simulink library "se2a_environment_lib"  (R2018b)
settings: Solver=VariableStepAuto  StartTime=0.0  StopTime=10.0  RelTol=1e-3
undefined symbols (not defined in the file or in its folder): aircraft, alt_ground, atmosphere, Atmosphere, cntrl, envir, g, ic, pos_ref, wind
libraries: simulink x9, atmosphere_lib x6, linear_systems_lib x6, $bdroot x5
(part 1 of 2)
settings Model: Creator=Ybeyer  LastModifiedBy=yannic
settings SFSimCC: SimUseLocalCustomCode=off
settings RTWCC: RTWUseLocalCustomCode=off
settings CodeAppCC: StateflowObjectComments=on

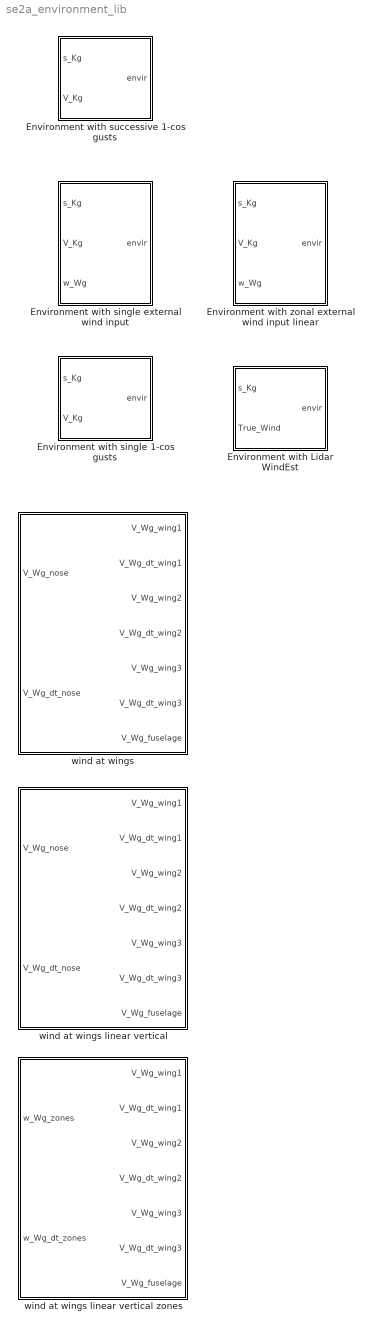
== system se2a_environment_lib ==
  Environment with Lidar WindEst : Subsystem  mask{envir=envir, pos_ref=pos_ref}
      mask prompts: envir "environment struct"; pos_ref "reference position struct"
      mask DialogControl DescGroupVar Prompt: Environment with successive 1-cos gusts
      mask DialogControl DescTextVar Prompt: Note that for the local gust delays the following structs must be in the base workspace: wing_main, wing_htp, wing_vtp, fuselage
  Environment with single 1-cos gusts : Subsystem  mask{envir=envir, pos_ref=pos_ref, wind_input=cntrl.wind_input, U_ds=-1, gust_dir=0, F_g=30, gustGradDist=30, Delta_gustGradDist=10, Delta_time=3, time_0=5}
      mask prompts: envir "environment struct"; pos_ref "reference position struct"; wind_input "Switch wing model (1=disable, 2=1-cos gust)"; U_ds "U_ds (Positive values only, if -1 value is calculated internally)"; gust_dir "Gust direction (>0 up, <0 down)"; F_g "Flight profile alleviation factor"; gustGradDist "Initial gust gradient distance, in ft"; Delta_gustGradDist "Delta gust gradient distance, in ft"; Delta_time "Time between gusts, in s"; time_0 "Time of first gust, in s"
      mask DialogControl DescGroupVar Prompt: Environment with successive 1-cos gusts
      mask DialogControl DescTextVar Prompt: Note that for the local gust delays the following structs must be in the base workspace: wing_main, wing_htp, wing_vtp, fuselage
  Environment with single external wind input : Subsystem  mask{aircraft=aircraft, V_A=norm(ic.V_Kb,2), pos_ref=pos_ref, k_max=1}
      mask prompts: aircraft "Aircraft parameters sturct, see aircraftSe2aCreate"; V_A "Airspeed (TAS) in m/s"; pos_ref "Reference position, see loadPosRef"; k_max "Wind derivative cutoff reduced frequency, rad"
      mask DialogControl DescGroupVar Prompt: Environment with single external wind input
      mask DialogControl Container2 Prompt: Parameters
  Environment with successive 1-cos gusts : Subsystem  mask{envir=envir, pos_ref=pos_ref, wind_input=cntrl.wind_input, F_g=1, gustGradDist=30, Delta_gustGradDist=10, Delta_time=3, time_0=5}
      mask prompts: envir "environment struct"; pos_ref "reference position struct"; wind_input "Switch wing model (1=disable, 2=1-cos gust)"; F_g "Flight profile alleviation factor"; gustGradDist "Initial gust gradient distance, in ft"; Delta_gustGradDist "Delta gust gradient distance, in ft"; Delta_time "Time between gusts, in s"; time_0 "Time of first gust, in s"
      mask DialogControl DescGroupVar Prompt: Environment with successive 1-cos gusts
      mask DialogControl DescTextVar Prompt: Note that for the local gust delays the following structs must be in the base workspace: wing_main, wing_htp, wing_vtp, fuselage
  Environment with zonal external wind input linear : Subsystem  mask{aircraft=aircraft, V_A=norm(ic.V_Kb,2), pos_ref=pos_ref, k_max=1}
      mask prompts: aircraft "Aircraft parameters sturct, see aircraftSe2aCreate"; V_A "Airspeed (TAS) in m/s"; pos_ref "Reference position, see loadPosRef"; k_max "Wind derivative cutoff reduced frequency, rad"
      mask DialogControl DescGroupVar Prompt: Environment with single external wind input
      mask DialogControl Container2 Prompt: Parameters
  wind at wings : Subsystem  mask{aircraft=aircraft, V_A=norm(ic.V_Kb,2)}
      mask prompts: aircraft "Aircraft parameters struct, see aircraftSe2aCreate"; V_A "Airspeed (TAS) in m/s"
      mask init:
      | Delta_time_main_wing = abs(aircraft.wing_main.params.x+aircraft.wing_main.geometry.ctrl_pt.pos(1,:))/V_A;
      | Delta_time_htp = abs(aircraft.wing_htp.params.x+aircraft.wing_htp.geometry.ctrl_pt.pos(1,:))/V_A;
      | Delta_time_vtp = abs(aircraft.wing_vtp.params.x+aircraft.wing_vtp.geometry.ctrl_pt.pos(1,:))/V_A;
      | Delta_time_fuse = abs(aircraft.fuselage.geometry.border_pos(1,:))/V_A;
  wind at wings linear vertical : Subsystem  mask{aircraft=aircraft, V_A=norm(ic.V_Kb,2)}
      mask prompts: aircraft "Aircraft parameters struct, see aircraftSe2aCreate"; V_A "Airspeed (TAS) in m/s"
      mask init:
      | Delta_time_main_wing = abs(aircraft.wing_main.params.x+aircraft.wing_main.geometry.ctrl_pt.pos(1,:))/V_A;
      | Delta_time_htp = abs(aircraft.wing_htp.params.x+aircraft.wing_htp.geometry.ctrl_pt.pos(1,:))/V_A;
      | Delta_time_vtp = abs(aircraft.wing_vtp.params.x+aircraft.wing_vtp.geometry.ctrl_pt.pos(1,:))/V_A;
      | Delta_time_fuse = abs(aircraft.fuselage.geometry.border_pos(1,:))/V_A;
      | 
      | Ts = 1/100;
      | 
      | Delay_sys_main_wing = Create_LinearDelaySys(Delta_time_main_wing, Ts);
      | Delay_sys_htp = Create_LinearDelaySys(Delta_time_htp, Ts);
      | Delay_sys_vtp = Create_LinearDelaySys(Delta_time_vtp, Ts);
      | Delay_sys_fuse = Create_LinearDelaySys(Delta_time_fuse, Ts);
  wind at wings linear vertical zones : Subsystem  mask{aircraft=aircraft, V_A=norm(ic.V_Kb,2)}
      mask prompts: aircraft "Aircraft parameters struct, see aircraftSe2aCreate"; V_A "Airspeed (TAS) in m/s"
      mask init:
      | Delta_time_main_wing = abs(aircraft.wing_main.params.x+aircraft.wing_main.geometry.ctrl_pt.pos(1,:))/V_A;
      | Delta_time_htp = abs(aircraft.wing_htp.params.x+aircraft.wing_htp.geometry.ctrl_pt.pos(1,:))/V_A;
      | Delta_time_vtp = abs(aircraft.wing_vtp.params.x+aircraft.wing_vtp.geometry.ctrl_pt.pos(1,:))/V_A;
      | Delta_time_fuse = abs(aircraft.fuselage.geometry.border_pos(1,:))/V_A;
      | 
      | Ts = 0;%1/100;
      | 
      | Delay_sys_main_wing = Create_LinearDelaySys(Delta_time_main_wing, Ts);
      | Delay_sys_htp = Create_LinearDelaySys(Delta_time_htp, Ts);
      | Delay_sys_vtp = Create_LinearDelaySys(Delta_time_vtp, Ts);
      | Delay_sys_fuse = Create_LinearDelaySys(Delta_time_fuse, Ts);

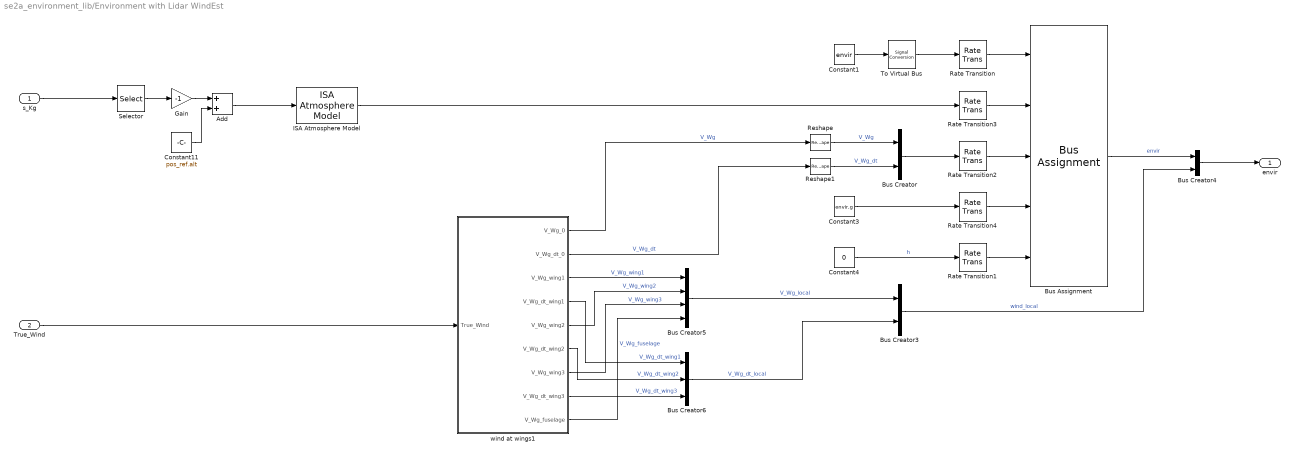
== system se2a_environment_lib/Environment with Lidar WindEst ==
  s_Kg : Inport
  True_Wind : Inport  Port=2
  Add : Sum
  Bus Assignment : BusAssignment  AssignedSignals=atmosphere,wind,g,alt_ground
  Bus Creator : BusCreator  Inputs=2
  Bus Creator3 : BusCreator  Inputs=2
  Bus Creator4 : BusCreator  Inputs=2
  Bus Creator5 : BusCreator  Inputs=4
  Bus Creator6 : BusCreator  Inputs=3
  Constant1 : Constant  Value=envir  OutDataTypeStr=Bus: envirBus
  Constant11 : Constant  Value=pos_ref.alt
  Constant3 : Constant  Value=envir.g
  Constant4 : Constant  Value=0
  Gain : Gain  Gain=-1
  ISA Atmosphere Model : atmosphere_lib/ISA Atmosphere Model
      settings: SourceProductName=LADAC
  Rate Transition{,1..4} (5 alike) : RateTransition
  Reshape : Reshape  OutputDimensionality=Column vector (2-D)
  Reshape1 : Reshape  OutputDimensionality=Column vector (2-D)
  Selector : Selector  InputPortWidth=3  IndexOptions=Index vector (dialog)  Indices=3  OutputSizes=1
  To Virtual Bus : SignalConversion  ConversionOutput=Virtual bus  OverrideOpt=off
  wind at wings1 : Subsystem  mask{aircraft=aircraft}
      mask prompts: aircraft "Aircraft parameters struct, see aircraftSe2aCreate"
      mask init:
      | n_origin = 6;
      | n_wing = aircraft.wing_main.n_panel;
      | n_htp = aircraft.wing_htp.n_panel;
      | n_vtp = aircraft.wing_vtp.n_panel;
      | n_fus = aircraft.fuselage.n_segments+1;
  envir : Outport
  wires:
  Constant4/1 -> Rate Transition1/1  "h"
  Rate Transition2/1 -> Bus Assignment/3
  Rate Transition3/1 -> Bus Assignment/2
  Bus Assignment/1 -> Bus Creator4/1  "envir"
  Rate Transition/1 -> Bus Assignment/1
  ISA Atmosphere Model/1 -> Rate Transition3/1
  Rate Transition1/1 -> Bus Assignment/5
  Constant1/1 -> To Virtual Bus/1
  Add/1 -> ISA Atmosphere Model/1
  Bus Creator/1 -> Rate Transition2/1
  wind at wings1/2(V_Wg_dt_0) -> Reshape1/1  "V_Wg_dt"
  Rate Transition4/1 -> Bus Assignment/4
  Constant3/1 -> Rate Transition4/1
  wind at wings1/1(V_Wg_0) -> Reshape/1  "V_Wg"
  Bus Creator6/1 -> Bus Creator3/2  "V_Wg_dt_local"
  Bus Creator3/1 -> Bus Creator4/2  "wind_local"
  Bus Creator4/1 -> envir/1
  To Virtual Bus/1 -> Rate Transition/1
  Constant11/1 -> Add/2
  Gain/1 -> Add/1
  s_Kg/1 -> Selector/1
  Selector/1 -> Gain/1
  True_Wind/1 -> wind at wings1/1(True_Wind)
  wind at wings1/8(V_Wg_dt_wing3) -> Bus Creator6/3  "V_Wg_dt_wing3"
  wind at wings1/6(V_Wg_dt_wing2) -> Bus Creator6/2  "V_Wg_dt_wing2"
  wind at wings1/5(V_Wg_wing2) -> Bus Creator5/2  "V_Wg_wing2"
  wind at wings1/9(V_Wg_fuselage) -> Bus Creator5/4  "V_Wg_fuselage"
  Bus Creator5/1 -> Bus Creator3/1  "V_Wg_local"
  wind at wings1/4(V_Wg_dt_wing1) -> Bus Creator6/1  "V_Wg_dt_wing1"
  wind at wings1/3(V_Wg_wing1) -> Bus Creator5/1  "V_Wg_wing1"
  wind at wings1/7(V_Wg_wing3) -> Bus Creator5/3  "V_Wg_wing3"
  Reshape/1 -> Bus Creator/1  "V_Wg"
  Reshape1/1 -> Bus Creator/2  "V_Wg_dt"

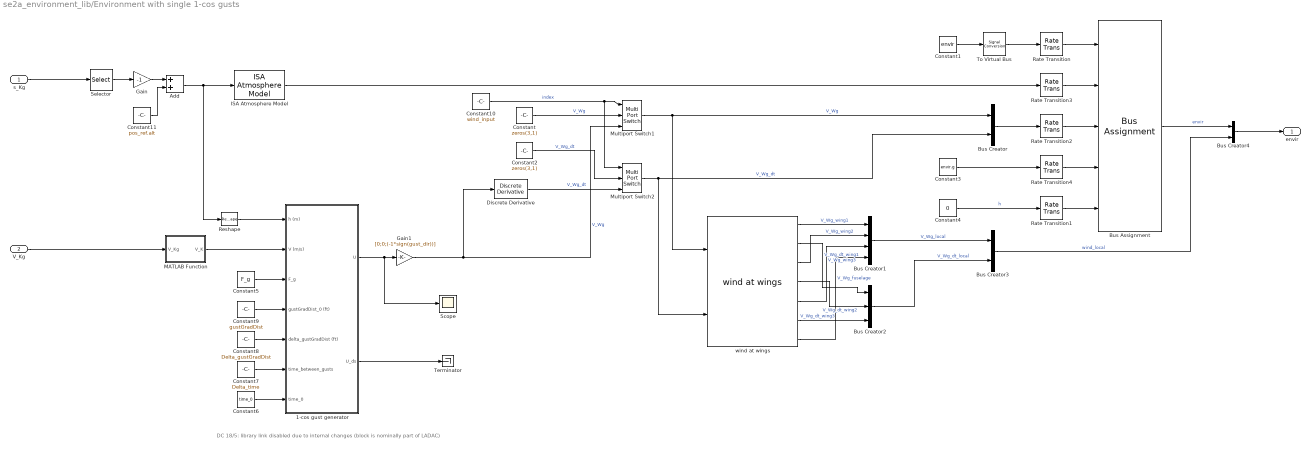
== system se2a_environment_lib/Environment with single 1-cos gusts ==
  note: DC 18/5: library link disabled due to internal changes (block is nominally part of LADAC)
  s_Kg : Inport
  V_Kg : Inport  Port=2
  1-cos gust generator : Subsystem  AncestorBlock=atmosphere_lib/1-cos gust generator
      mask DialogControl DescGroupVar Prompt: 1-cos gust generator
      mask DialogControl DescTextVar Prompt: With this block you can generate a time series of 1-cos gusts. You can use the inputs to specify parameters like the initial gust gradient distance and how you want to increment the gust gradient distance for the next gust. Moreover, you can specify the time between the gusts.
      mask DialogControl ParameterGroupVar Prompt: Inputs
      mask DialogControl Control2 Prompt: h - altitude (m)
      mask DialogControl Control3 Prompt: V - airspeed of the aircraft (m/s)
      mask DialogControl Control4 Prompt: F_g - flight profile alleviation factor
      mask DialogControl Control5 Prompt: gustGradDist_0 - initial gust gradient distance (m)
      mask DialogControl Control6 Prompt: delta_gustGradDist - difference of the gust gradient distance for the next gust (m)
      mask DialogControl Control7 Prompt: time_between gusts - the time between gusts where there will be no wind (s)
      mask DialogControl Control8 Prompt: time_0 - time when the first gust starts
  Add : Sum
  Bus Assignment : BusAssignment  AssignedSignals=atmosphere,wind,g,alt_ground
  Bus Creator : BusCreator  Inputs=2
  Bus Creator1 : BusCreator  Inputs=4
  Bus Creator2 : BusCreator  Inputs=3
  Bus Creator3 : BusCreator  Inputs=2
  Bus Creator4 : BusCreator  Inputs=2
  Constant : Constant  Value=zeros(3,1)  VectorParams1D=off
  Constant1 : Constant  Value=envir  OutDataTypeStr=Bus: envirBus
  Constant10 : Constant  Value=wind_input
  Constant11 : Constant  Value=pos_ref.alt
  Constant2 : Constant  Value=zeros(3,1)  VectorParams1D=off
  Constant3 : Constant  Value=envir.g
  Constant4 : Constant  Value=0
  Constant5 : Constant  Value=F_g
  Constant6 : Constant  Value=time_0
  Constant7 : Constant  Value=Delta_time
  Constant8 : Constant  Value=Delta_gustGradDist
  Constant9 : Constant  Value=gustGradDist
  Discrete Derivative : simulink/Discrete/Discrete Derivative  gainval=1.0  ICPrevScaledInput=0.0  OutMin=[]  OutMax=[]  OutDataType=fixdt(1, 16)  OutScaling=2^-10  DoSatur=off
  Gain : Gain  Gain=-1
  Gain1 : Gain  Gain=[0;0;(-1*sign(gust_dir))]
  ISA Atmosphere Model : atmosphere_lib/ISA Atmosphere Model
      settings: SourceProductName=LADAC
  MATLAB Function : MATLAB Function  TreatAsAtomicUnit=on
  Multiport Switch1 : MultiPortSwitch  Inputs=2
  Multiport Switch2 : MultiPortSwitch  Inputs=2
  Rate Transition{,1..4} (5 alike) : RateTransition
  Reshape : Reshape
  Scope : Scope
  Selector : Selector  InputPortWidth=3  IndexOptions=Index vector (dialog)  Indices=3  OutputSizes=1
  Terminator : Terminator
  To Virtual Bus : SignalConversion  ConversionOutput=Virtual bus  OverrideOpt=off
  wind at wings : $bdroot/wind at wings  aircraft=aircraft  V_A=norm(ic.V_Kb,2)
  envir : Outport
  wires:
  Reshape/1 -> 1-cos gust generator/1(h (m))
  wind at wings/7 -> Bus Creator1/4  "V_Wg_fuselage"
  Selector/1 -> Gain/1
  s_Kg/1 -> Selector/1
  Gain/1 -> Add/1
  Constant11/1 -> Add/2
  To Virtual Bus/1 -> Rate Transition/1
  Bus Creator4/1 -> envir/1
  Bus Creator3/1 -> Bus Creator4/2  "wind_local"
  Bus Creator2/1 -> Bus Creator3/2  "V_Wg_dt_local"
  wind at wings/2 -> Bus Creator2/1  "V_Wg_dt_wing1"
  wind at wings/4 -> Bus Creator2/2  "V_Wg_dt_wing2"
  wind at wings/6 -> Bus Creator2/3  "V_Wg_dt_wing3"
  Bus Creator1/1 -> Bus Creator3/1  "V_Wg_local"
  wind at wings/5 -> Bus Creator1/3  "V_Wg_wing3"
  wind at wings/3 -> Bus Creator1/2  "V_Wg_wing2"
  wind at wings/1 -> Bus Creator1/1  "V_Wg_wing1"
  Discrete Derivative/1 -> Multiport Switch2/3  "V_Wg_dt"
  Constant2/1 -> Multiport Switch2/2  "V_Wg_dt"
  Constant10/1 -> Multiport Switch1/1, Multiport Switch2/1  "index"
  Multiport Switch1/1 -> wind at wings/1, Bus Creator/1  "V_Wg"
  Constant/1 -> Multiport Switch1/2  "V_Wg"
  1-cos gust generator/2(U_ds) -> Terminator/1
  1-cos gust generator/1(U) -> Scope/1, Gain1/1
  MATLAB Function/1(V_K) -> 1-cos gust generator/2(V (m/s))
  Constant9/1 -> 1-cos gust generator/4(gustGradDist_0 (ft))
  Constant8/1 -> 1-cos gust generator/5(delta_gustGradDist (ft))
  Constant7/1 -> 1-cos gust generator/6(time_between_gusts)
  Constant6/1 -> 1-cos gust generator/7(time_0)
  Constant5/1 -> 1-cos gust generator/3(F_g)
  Constant3/1 -> Rate Transition4/1
  Rate Transition4/1 -> Bus Assignment/4
  Multiport Switch2/1 -> wind at wings/2, Bus Creator/2  "V_Wg_dt"
  Bus Creator/1 -> Rate Transition2/1
  Add/1 -> ISA Atmosphere Model/1, Reshape/1
  Constant1/1 -> To Virtual Bus/1
  Rate Transition1/1 -> Bus Assignment/5
  ISA Atmosphere Model/1 -> Rate Transition3/1
  Rate Transition/1 -> Bus Assignment/1
  Bus Assignment/1 -> Bus Creator4/1  "envir"
  Rate Transition3/1 -> Bus Assignment/2
  Rate Transition2/1 -> Bus Assignment/3
  Constant4/1 -> Rate Transition1/1  "h"
  V_Kg/1 -> MATLAB Function/1(V_Kg)
  Gain1/1 -> Multiport Switch1/3, Discrete Derivative/1  "V_Wg"

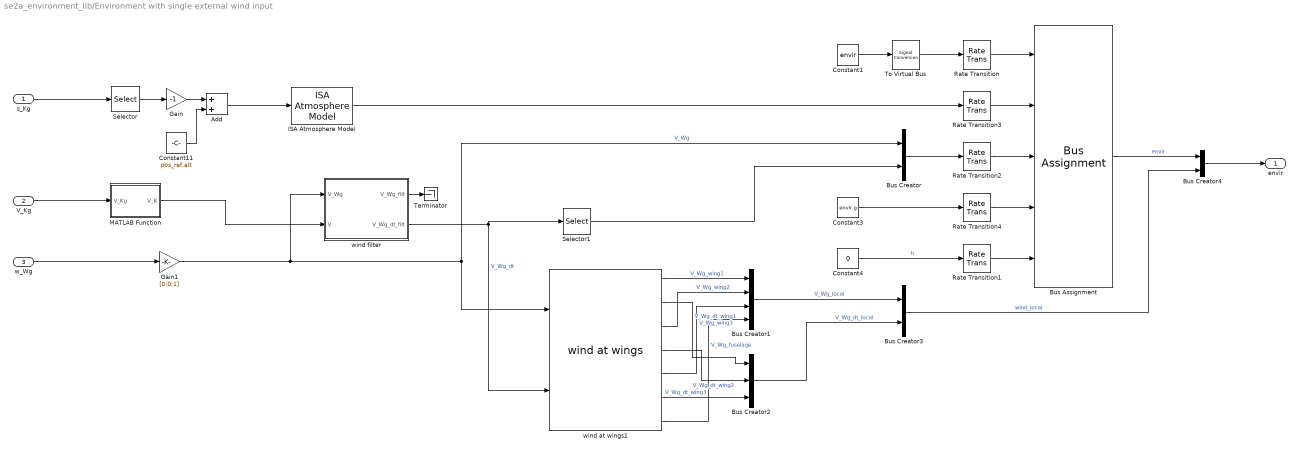
== system se2a_environment_lib/Environment with single external wind input ==
  s_Kg : Inport
  V_Kg : Inport  Port=2
  w_Wg : Inport  Port=3
  Add : Sum
  Bus Assignment : BusAssignment  AssignedSignals=atmosphere,wind,g,alt_ground
  Bus Creator : BusCreator  Inputs=2
  Bus Creator1 : BusCreator  Inputs=4
  Bus Creator2 : BusCreator  Inputs=3
  Bus Creator3 : BusCreator  Inputs=2
  Bus Creator4 : BusCreator  Inputs=2
  Constant1 : Constant  Value=envir  OutDataTypeStr=Bus: envirBus
  Constant11 : Constant  Value=pos_ref.alt
  Constant3 : Constant  Value=envir.g
  Constant4 : Constant  Value=0
  Gain : Gain  Gain=-1
  Gain1 : Gain  Gain=[0;0;1]
  ISA Atmosphere Model : atmosphere_lib/ISA Atmosphere Model
      settings: SourceProductName=LADAC
  MATLAB Function : MATLAB Function  TreatAsAtomicUnit=on
  Rate Transition{,1..4} (5 alike) : RateTransition
  Selector : Selector  InputPortWidth=3  IndexOptions=Index vector (dialog)  Indices=3  OutputSizes=1
  Selector1 : Selector  NumberOfDimensions=2  InputPortWidth=3  IndexOptions=Index vector (dialog),Index vector (dialog)  Indices=1:3,1  OutputSizes=1,1
  Terminator : Terminator
  To Virtual Bus : SignalConversion  ConversionOutput=Virtual bus  OverrideOpt=off
  wind at wings1 : $bdroot/wind at wings  aircraft=aircraft  V_A=V_A
  wind filter : Subsystem
  envir : Outport
  wires:
  s_Kg/1 -> Selector/1
  Selector/1 -> Gain/1
  Constant11/1 -> Add/2
  Add/1 -> ISA Atmosphere Model/1
  Gain/1 -> Add/1
  Constant1/1 -> To Virtual Bus/1
  wind at wings1/7 -> Bus Creator1/4  "V_Wg_fuselage"
  wind at wings1/3 -> Bus Creator1/2  "V_Wg_wing2"
  Bus Creator1/1 -> Bus Creator3/1  "V_Wg_local"
  Rate Transition3/1 -> Bus Assignment/2
  wind at wings1/1 -> Bus Creator1/1  "V_Wg_wing1"
  wind filter/2(V_Wg_dt_filt) -> wind at wings1/2, Selector1/1  "V_Wg_dt"
  Constant3/1 -> Rate Transition4/1
  Constant4/1 -> Rate Transition1/1  "h"
  Rate Transition4/1 -> Bus Assignment/4
  Rate Transition/1 -> Bus Assignment/1
  Bus Assignment/1 -> Bus Creator4/1  "envir"
  Rate Transition1/1 -> Bus Assignment/5
  Rate Transition2/1 -> Bus Assignment/3
  wind at wings1/2 -> Bus Creator2/1  "V_Wg_dt_wing1"
  To Virtual Bus/1 -> Rate Transition/1
  Bus Creator2/1 -> Bus Creator3/2  "V_Wg_dt_local"
  Bus Creator/1 -> Rate Transition2/1
  Bus Creator4/1 -> envir/1
  wind at wings1/6 -> Bus Creator2/3  "V_Wg_dt_wing3"
  ISA Atmosphere Model/1 -> Rate Transition3/1
  Gain1/1 -> wind filter/1(V_Wg), Bus Creator/1, wind at wings1/1  "V_Wg"
  Bus Creator3/1 -> Bus Creator4/2  "wind_local"
  wind at wings1/5 -> Bus Creator1/3  "V_Wg_wing3"
  wind at wings1/4 -> Bus Creator2/2  "V_Wg_dt_wing2"
  w_Wg/1 -> Gain1/1
  wind filter/1(V_Wg_filt) -> Terminator/1
  MATLAB Function/1(V_K) -> wind filter/2(V)
  V_Kg/1 -> MATLAB Function/1(V_Kg)
  Selector1/1 -> Bus Creator/2

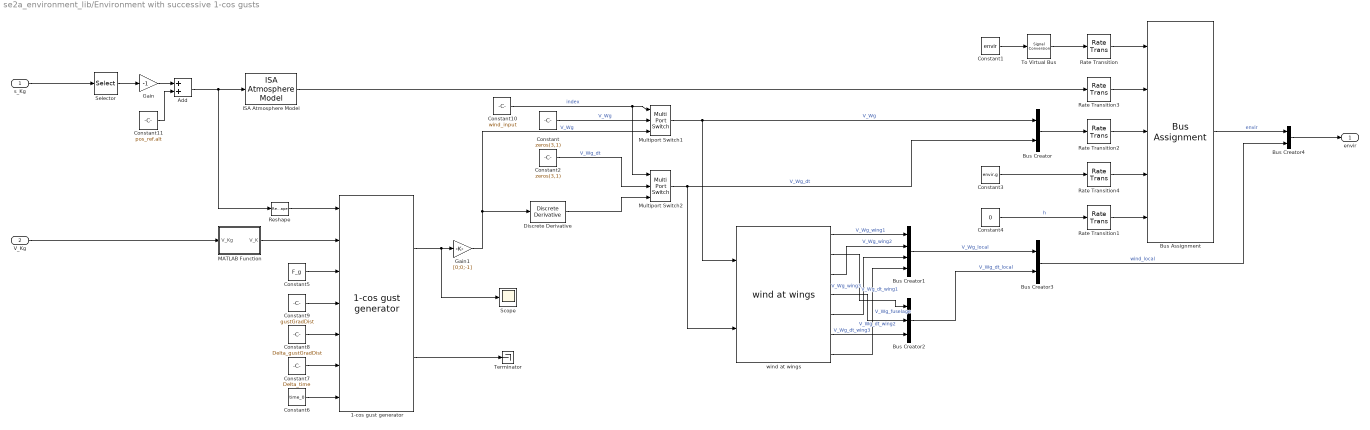
== system se2a_environment_lib/Environment with successive 1-cos gusts ==
  s_Kg : Inport
  V_Kg : Inport  Port=2
  1-cos gust generator : atmosphere_lib/1-cos gust generator
      settings: SourceProductName=LADAC
  Add : Sum
  Bus Assignment : BusAssignment  AssignedSignals=atmosphere,wind,g,alt_ground
  Bus Creator : BusCreator  Inputs=2
  Bus Creator1 : BusCreator  Inputs=4
  Bus Creator2 : BusCreator  Inputs=3
  Bus Creator3 : BusCreator  Inputs=2
  Bus Creator4 : BusCreator  Inputs=2
  Constant : Constant  Value=zeros(3,1)  VectorParams1D=off
  Constant1 : Constant  Value=envir  OutDataTypeStr=Bus: envirBus
  Constant10 : Constant  Value=wind_input
  Constant11 : Constant  Value=pos_ref.alt
  Constant2 : Constant  Value=zeros(3,1)  VectorParams1D=off
  Constant3 : Constant  Value=envir.g
  Constant4 : Constant  Value=0
  Constant5 : Constant  Value=F_g
  Constant6 : Constant  Value=time_0
  Constant7 : Constant  Value=Delta_time
  Constant8 : Constant  Value=Delta_gustGradDist
  Constant9 : Constant  Value=gustGradDist
  Discrete Derivative : simulink/Discrete/Discrete Derivative  gainval=1.0  ICPrevScaledInput=0.0  OutMin=[]  OutMax=[]  OutDataType=fixdt(1, 16)  OutScaling=2^-10  DoSatur=off
  Gain : Gain  Gain=-1
  Gain1 : Gain  Gain=[0;0;-1]
  ISA Atmosphere Model : atmosphere_lib/ISA Atmosphere Model
      settings: SourceProductName=LADAC
  MATLAB Function : MATLAB Function  TreatAsAtomicUnit=on
  Multiport Switch1 : MultiPortSwitch  Inputs=2
  Multiport Switch2 : MultiPortSwitch  Inputs=2
  Rate Transition{,1..4} (5 alike) : RateTransition
  Reshape : Reshape
  Scope : Scope
  Selector : Selector  InputPortWidth=3  IndexOptions=Index vector (dialog)  Indices=3  OutputSizes=1
  Terminator : Terminator
  To Virtual Bus : SignalConversion  ConversionOutput=Virtual bus  OverrideOpt=off
  wind at wings : $bdroot/wind at wings  aircraft=aircraft  V_A=norm(ic.V_Kb,2)
  envir : Outport
  wires:
  Constant4/1 -> Rate Transition1/1  "h"
  Rate Transition2/1 -> Bus Assignment/3
  Rate Transition3/1 -> Bus Assignment/2
  Bus Assignment/1 -> Bus Creator4/1  "envir"
  Rate Transition/1 -> Bus Assignment/1
  ISA Atmosphere Model/1 -> Rate Transition3/1
  Rate Transition1/1 -> Bus Assignment/5
  Constant1/1 -> To Virtual Bus/1
  Add/1 -> Reshape/1, ISA Atmosphere Model/1
  Bus Creator/1 -> Rate Transition2/1
  Multiport Switch2/1 -> wind at wings/2, Bus Creator/2  "V_Wg_dt"
  Rate Transition4/1 -> Bus Assignment/4
  Constant3/1 -> Rate Transition4/1
  Constant5/1 -> 1-cos gust generator/3
  Constant6/1 -> 1-cos gust generator/7
  Constant7/1 -> 1-cos gust generator/6
  Constant8/1 -> 1-cos gust generator/5
  Constant9/1 -> 1-cos gust generator/4
  V_Kg/1 -> MATLAB Function/1(V_Kg)
  MATLAB Function/1(V_K) -> 1-cos gust generator/2
  1-cos gust generator/1 -> Gain1/1, Scope/1
  1-cos gust generator/2 -> Terminator/1
  Constant/1 -> Multiport Switch1/2  "V_Wg"
  Multiport Switch1/1 -> wind at wings/1, Bus Creator/1  "V_Wg"
  Constant10/1 -> Multiport Switch2/1, Multiport Switch1/1  "index"
  Gain1/1 -> Discrete Derivative/1, Multiport Switch1/3  "V_Wg"
  Constant2/1 -> Multiport Switch2/2  "V_Wg_dt"
  wind at wings/1 -> Bus Creator1/1  "V_Wg_wing1"
  wind at wings/3 -> Bus Creator1/2  "V_Wg_wing2"
  wind at wings/5 -> Bus Creator1/3  "V_Wg_wing3"
  Bus Creator1/1 -> Bus Creator3/1  "V_Wg_local"
  wind at wings/6 -> Bus Creator2/3  "V_Wg_dt_wing3"
  wind at wings/4 -> Bus Creator2/2  "V_Wg_dt_wing2"
  wind at wings/2 -> Bus Creator2/1  "V_Wg_dt_wing1"
  Bus Creator2/1 -> Bus Creator3/2  "V_Wg_dt_local"
  Bus Creator3/1 -> Bus Creator4/2  "wind_local"
  Bus Creator4/1 -> envir/1
  To Virtual Bus/1 -> Rate Transition/1
  Constant11/1 -> Add/2
  Gain/1 -> Add/1
  s_Kg/1 -> Selector/1
  Selector/1 -> Gain/1
  wind at wings/7 -> Bus Creator1/4  "V_Wg_fuselage"
  Reshape/1 -> 1-cos gust generator/1
  Discrete Derivative/1 -> Multiport Switch2/3

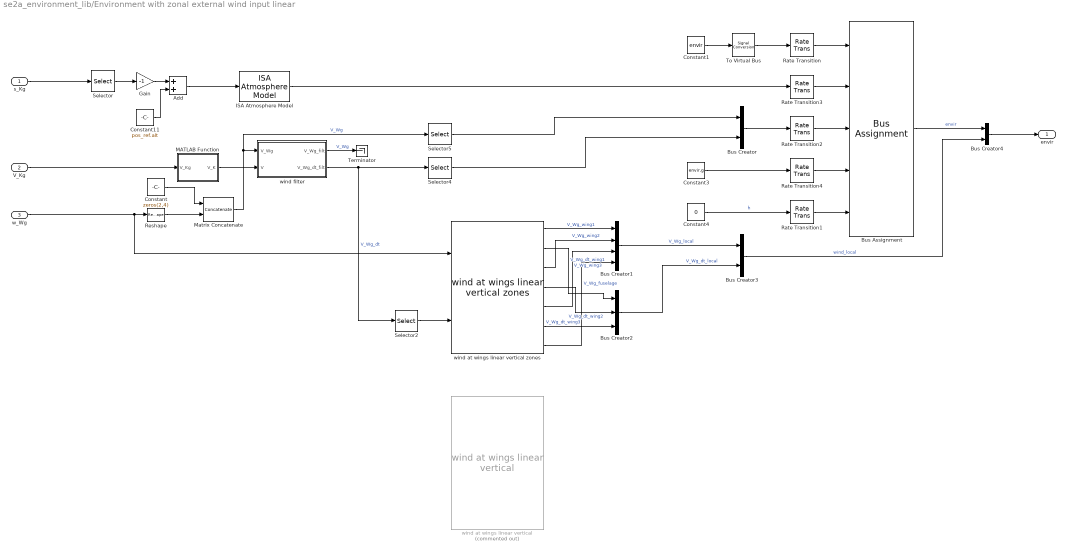
== system se2a_environment_lib/Environment with zonal external wind input linear ==
  s_Kg : Inport
  V_Kg : Inport  Port=2
  w_Wg : Inport  Port=3
  Add : Sum
  Bus Assignment : BusAssignment  AssignedSignals=atmosphere,wind,g,alt_ground
  Bus Creator : BusCreator  Inputs=2
  Bus Creator1 : BusCreator  Inputs=4
  Bus Creator2 : BusCreator  Inputs=3
  Bus Creator3 : BusCreator  Inputs=2
  Bus Creator4 : BusCreator  Inputs=2
  Constant : Constant  Value=zeros(2,4)
  Constant1 : Constant  Value=envir  OutDataTypeStr=Bus: envirBus
  Constant11 : Constant  Value=pos_ref.alt
  Constant3 : Constant  Value=envir.g
  Constant4 : Constant  Value=0
  Gain : Gain  Gain=-1
  ISA Atmosphere Model : atmosphere_lib/ISA Atmosphere Model
      settings: SourceProductName=LADAC
  MATLAB Function : MATLAB Function  TreatAsAtomicUnit=on
  Matrix Concatenate : Concatenate  Mode=Multidimensional array
  Rate Transition{,1..4} (5 alike) : RateTransition
  Reshape : Reshape  OutputDimensionality=Row vector (2-D)
  Selector : Selector  InputPortWidth=3  IndexOptions=Index vector (dialog)  Indices=3  OutputSizes=1
  Selector2 : Selector  NumberOfDimensions=2  InputPortWidth=4  IndexOptions=Index vector (dialog),Select all  Indices=3,1  OutputSizes=1,1
  Selector4 : Selector  NumberOfDimensions=2  InputPortWidth=4  IndexOptions=Index vector (dialog),Index vector (dialog)  Indices=1:3,4  OutputSizes=1,1
  Selector5 : Selector  NumberOfDimensions=2  InputPortWidth=4  IndexOptions=Index vector (dialog),Index vector (dialog)  Indices=1:3,4  OutputSizes=1,1
  Terminator : Terminator
  To Virtual Bus : SignalConversion  ConversionOutput=Virtual bus  OverrideOpt=off
  wind at wings linear vertical : $bdroot/wind at wings linear vertical  Commented=on  aircraft=aircraft  V_A=norm(ic.V_Kb,2)
  wind at wings linear vertical zones : $bdroot/wind at wings linear vertical zones  aircraft=aircraft  V_A=norm(ic.V_Kb,2)
  wind filter : Subsystem
  envir : Outport
  wires:
  s_Kg/1 -> Selector/1
  Selector/1 -> Gain/1
  Constant11/1 -> Add/2
  Add/1 -> ISA Atmosphere Model/1
  Gain/1 -> Add/1
  Constant1/1 -> To Virtual Bus/1
  wind at wings linear vertical zones/7 -> Bus Creator1/4  "V_Wg_fuselage"
  wind at wings linear vertical zones/3 -> Bus Creator1/2  "V_Wg_wing2"
  Bus Creator1/1 -> Bus Creator3/1  "V_Wg_local"
  Rate Transition3/1 -> Bus Assignment/2
  wind at wings linear vertical zones/1 -> Bus Creator1/1  "V_Wg_wing1"
  wind filter/2(V_Wg_dt_filt) -> Selector4/1, Selector2/1  "V_Wg_dt"
  Constant3/1 -> Rate Transition4/1
  Constant4/1 -> Rate Transition1/1  "h"
  Rate Transition4/1 -> Bus Assignment/4
  Rate Transition/1 -> Bus Assignment/1
  Bus Assignment/1 -> Bus Creator4/1  "envir"
  Rate Transition1/1 -> Bus Assignment/5
  Rate Transition2/1 -> Bus Assignment/3
  wind at wings linear vertical zones/2 -> Bus Creator2/1  "V_Wg_dt_wing1"
  To Virtual Bus/1 -> Rate Transition/1
  Bus Creator2/1 -> Bus Creator3/2  "V_Wg_dt_local"
  Bus Creator/1 -> Rate Transition2/1
  Bus Creator4/1 -> envir/1
  wind at wings linear vertical zones/6 -> Bus Creator2/3  "V_Wg_dt_wing3"
  ISA Atmosphere Model/1 -> Rate Transition3/1
  Bus Creator3/1 -> Bus Creator4/2  "wind_local"
  wind at wings linear vertical zones/5 -> Bus Creator1/3  "V_Wg_wing3"
  wind at wings linear vertical zones/4 -> Bus Creator2/2  "V_Wg_dt_wing2"
  V_Kg/1 -> MATLAB Function/1(V_Kg)
  wind filter/1(V_Wg_filt) -> Terminator/1  "V_Wg"
  MATLAB Function/1(V_K) -> wind filter/2(V)
  w_Wg/1 -> Reshape/1, wind at wings linear vertical zones/1
  Selector4/1 -> Bus Creator/2
  Selector5/1 -> Bus Creator/1
  Constant/1 -> Matrix Concatenate/1
  Reshape/1 -> Matrix Concatenate/2
  Matrix Concatenate/1 -> wind filter/1(V_Wg), Selector5/1  "V_Wg"
  Selector2/1 -> wind at wings linear vertical zones/2

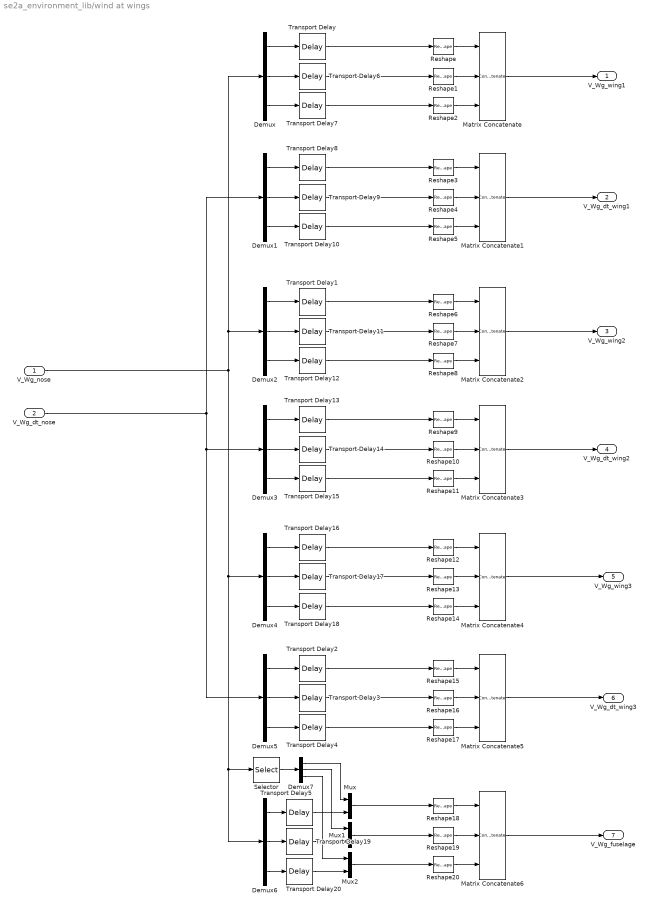
== system se2a_environment_lib/wind at wings ==
  V_Wg_nose : Inport
  V_Wg_dt_nose : Inport  Port=2
  Demux{,1..7} (8 alike) : Demux  Outputs=3
  Matrix Concatenate{,1..6} (7 alike) : Concatenate  NumInputs=3  Mode=Multidimensional array
  Mux : Mux  Inputs=2
  Mux1 : Mux  Inputs=2
  Mux2 : Mux  Inputs=2
  Reshape{,1..20} (21 alike) : Reshape  OutputDimensionality=Row vector (2-D)
  Selector : Selector  NumberOfDimensions=2  InputPortWidth=3  IndexOptions=Index vector (dialog),Index vector (dialog)  Indices=1:3,1  OutputSizes=1,1
  Transport Delay{,6..10} (6 alike) : TransportDelay  DelayTime=Delta_time_main_wing
  Transport Delay{1,11..15} (6 alike) : TransportDelay  DelayTime=Delta_time_htp
  Transport Delay{2..4,16..18} (6 alike) : TransportDelay  DelayTime=Delta_time_vtp
  Transport Delay19 : TransportDelay  DelayTime=Delta_time_fuse(2:end)
  Transport Delay20 : TransportDelay  DelayTime=Delta_time_fuse(2:end)
  Transport Delay5 : TransportDelay  DelayTime=Delta_time_fuse(2:end)
  V_Wg_wing1 : Outport
  V_Wg_dt_wing1 : Outport  Port=2
  V_Wg_wing2 : Outport  Port=3
  V_Wg_dt_wing2 : Outport  Port=4
  V_Wg_wing3 : Outport  Port=5
  V_Wg_dt_wing3 : Outport  Port=6
  V_Wg_fuselage : Outport  Port=7
  wires:
  Demux7/3 -> Mux2/1
  Demux7/2 -> Mux1/1
  Demux7/1 -> Mux/1
  Selector/1 -> Demux7/1
  Mux2/1 -> Reshape20/1
  Mux1/1 -> Reshape19/1
  Mux/1 -> Reshape18/1
  Demux6/2 -> Transport Delay19/1
  Transport Delay19/1 -> Mux1/2
  Transport Delay5/1 -> Mux/2
  Demux6/1 -> Transport Delay5/1
  Demux6/3 -> Transport Delay20/1
  Transport Delay20/1 -> Mux2/2
  Matrix Concatenate6/1 -> V_Wg_fuselage/1
  Matrix Concatenate5/1 -> V_Wg_dt_wing3/1
  Transport Delay4/1 -> Reshape17/1
  Demux5/3 -> Transport Delay4/1
  Demux5/1 -> Transport Delay2/1
  Transport Delay2/1 -> Reshape15/1
  Transport Delay3/1 -> Reshape16/1
  Demux5/2 -> Transport Delay3/1
  Matrix Concatenate4/1 -> V_Wg_wing3/1
  Transport Delay16/1 -> Reshape12/1
  Transport Delay17/1 -> Reshape13/1
  Transport Delay18/1 -> Reshape14/1
  Demux4/3 -> Transport Delay18/1
  Demux4/2 -> Transport Delay17/1
  Demux4/1 -> Transport Delay16/1
  Matrix Concatenate3/1 -> V_Wg_dt_wing2/1
  Demux3/1 -> Transport Delay13/1
  Demux3/2 -> Transport Delay14/1
  Demux3/3 -> Transport Delay15/1
  Transport Delay15/1 -> Reshape11/1
  Transport Delay14/1 -> Reshape10/1
  Transport Delay13/1 -> Reshape9/1
  Matrix Concatenate2/1 -> V_Wg_wing2/1
  Transport Delay1/1 -> Reshape6/1
  Transport Delay11/1 -> Reshape7/1
  Transport Delay12/1 -> Reshape8/1
  Demux2/3 -> Transport Delay12/1
  Demux2/2 -> Transport Delay11/1
  Demux2/1 -> Transport Delay1/1
  Transport Delay8/1 -> Reshape3/1
  Matrix Concatenate1/1 -> V_Wg_dt_wing1/1
  Demux1/1 -> Transport Delay8/1
  Demux1/3 -> Transport Delay10/1
  Transport Delay9/1 -> Reshape4/1
  Transport Delay10/1 -> Reshape5/1
  Demux1/2 -> Transport Delay9/1
  Transport Delay/1 -> Reshape/1
  Matrix Concatenate/1 -> V_Wg_wing1/1
  Transport Delay7/1 -> Reshape2/1
  Transport Delay6/1 -> Reshape1/1
  Demux/3 -> Transport Delay7/1
  Demux/2 -> Transport Delay6/1
  Demux/1 -> Transport Delay/1
  V_Wg_dt_nose/1 -> Demux1/1, Demux3/1, Demux5/1
  V_Wg_nose/1 -> Demux4/1, Demux6/1, Selector/1, Demux/1, Demux2/1
  Reshape/1 -> Matrix Concatenate/1
  Reshape1/1 -> Matrix Concatenate/2
  Reshape2/1 -> Matrix Concatenate/3
  Reshape3/1 -> Matrix Concatenate1/1
  Reshape4/1 -> Matrix Concatenate1/2
  Reshape5/1 -> Matrix Concatenate1/3
  Reshape6/1 -> Matrix Concatenate2/1
  Reshape7/1 -> Matrix Concatenate2/2
  Reshape8/1 -> Matrix Concatenate2/3
  Reshape9/1 -> Matrix Concatenate3/1
  Reshape10/1 -> Matrix Concatenate3/2
  Reshape11/1 -> Matrix Concatenate3/3
  Reshape12/1 -> Matrix Concatenate4/1
  Reshape13/1 -> Matrix Concatenate4/2
  Reshape14/1 -> Matrix Concatenate4/3
  Reshape15/1 -> Matrix Concatenate5/1
  Reshape16/1 -> Matrix Concatenate5/2
  Reshape17/1 -> Matrix Concatenate5/3
  Reshape18/1 -> Matrix Concatenate6/1
  Reshape19/1 -> Matrix Concatenate6/2
  Reshape20/1 -> Matrix Concatenate6/3

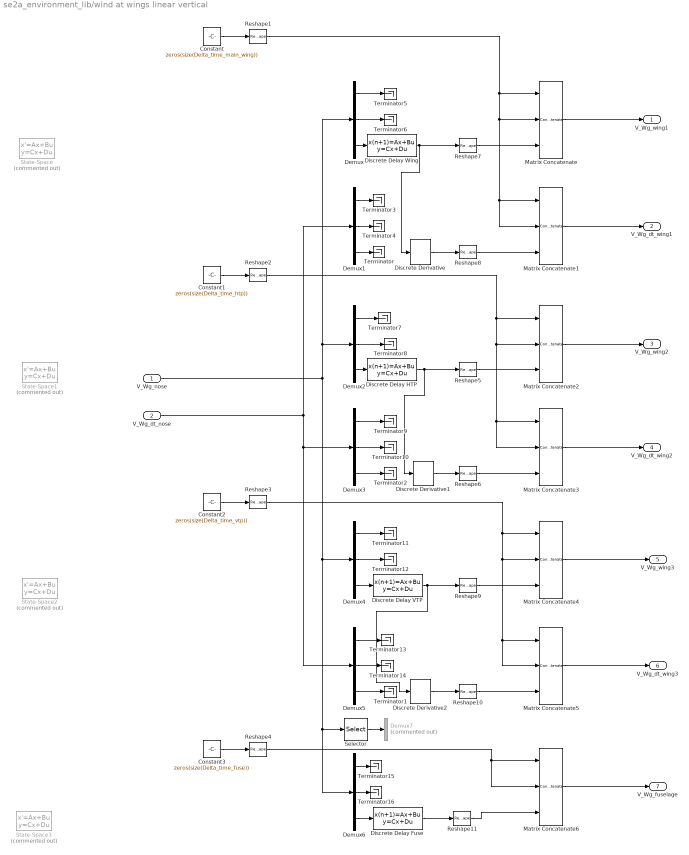
== system se2a_environment_lib/wind at wings linear vertical ==
  V_Wg_nose : Inport
  V_Wg_dt_nose : Inport  Port=2
  Constant : Constant  Value=zeros(size(Delta_time_main_wing))
  Constant1 : Constant  Value=zeros(size(Delta_time_htp))
  Constant2 : Constant  Value=zeros(size(Delta_time_vtp))
  Constant3 : Constant  Value=zeros(size(Delta_time_fuse))
  Demux{,1..6} (7 alike) : Demux  Outputs=3
  Demux7 : Demux  Commented=on  Outputs=3
  Discrete Delay Fuse : DiscreteStateSpace  A=Delay_sys_fuse.A  B=Delay_sys_fuse.B  C=Delay_sys_fuse.C  D=Delay_sys_fuse.D  SampleTime=Delay_sys_fuse.Ts
  Discrete Delay HTP : DiscreteStateSpace  A=Delay_sys_htp.A  B=Delay_sys_htp.B  C=Delay_sys_htp.C  D=Delay_sys_htp.D  SampleTime=Delay_sys_htp.Ts
  Discrete Delay VTP : DiscreteStateSpace  A=Delay_sys_vtp.A  B=Delay_sys_vtp.B  C=Delay_sys_vtp.C  D=Delay_sys_vtp.D  SampleTime=Delay_sys_vtp.Ts
  Discrete Delay Wing : DiscreteStateSpace  A=Delay_sys_main_wing.A  B=Delay_sys_main_wing.B  C=Delay_sys_main_wing.C  D=Delay_sys_main_wing.D  SampleTime=Delay_sys_main_wing.Ts
  Discrete Derivative : simulink/Discrete/Discrete Derivative  gainval=1.0  ICPrevScaledInput=0.0  OutMin=[]  OutMax=[]  OutDataType=fixdt(1, 16)  OutScaling=2^-10  DoSatur=off
  Discrete Derivative1 : simulink/Discrete/Discrete Derivative  gainval=1.0  ICPrevScaledInput=0.0  OutMin=[]  OutMax=[]  OutDataType=fixdt(1, 16)  OutScaling=2^-10  DoSatur=off
  Discrete Derivative2 : simulink/Discrete/Discrete Derivative  gainval=1.0  ICPrevScaledInput=0.0  OutMin=[]  OutMax=[]  OutDataType=fixdt(1, 16)  OutScaling=2^-10  DoSatur=off
  Matrix Concatenate{,1..6} (7 alike) : Concatenate  NumInputs=3  Mode=Multidimensional array
  Reshape{1..11} (11 alike) : Reshape  OutputDimensionality=Row vector (2-D)
  Selector : Selector  NumberOfDimensions=2  InputPortWidth=3  IndexOptions=Index vector (dialog),Index vector (dialog)  Indices=1:3,1  OutputSizes=1,1
  State-Space : StateSpace  Commented=on  A=Delay_sys_main_wing.A  B=Delay_sys_main_wing.B  C=Delay_sys_main_wing.C  D=Delay_sys_main_wing.D  InitialCondition=0
  State-Space1 : StateSpace  Commented=on  A=Delay_sys_htp.A  B=Delay_sys_htp.B  C=Delay_sys_htp.C  D=Delay_sys_htp.D  InitialCondition=0
  State-Space2 : StateSpace  Commented=on  A=Delay_sys_vtp.A  B=Delay_sys_vtp.B  C=Delay_sys_vtp.C  D=Delay_sys_vtp.D  InitialCondition=0
  State-Space3 : StateSpace  Commented=on  A=Delay_sys_fuse.A  B=Delay_sys_fuse.B  C=Delay_sys_fuse.C  D=Delay_sys_fuse.D  InitialCondition=0
  Terminator{,1..16} (17 alike) : Terminator
  V_Wg_wing1 : Outport
  V_Wg_dt_wing1 : Outport  Port=2
  V_Wg_wing2 : Outport  Port=3
  V_Wg_dt_wing2 : Outport  Port=4
  V_Wg_wing3 : Outport  Port=5
  V_Wg_dt_wing3 : Outport  Port=6
  V_Wg_fuselage : Outport  Port=7
  wires:
  V_Wg_nose/1 -> Demux2/1, Demux/1, Selector/1, Demux6/1, Demux4/1
  V_Wg_dt_nose/1 -> Demux5/1, Demux3/1, Demux1/1
  Demux/1 -> Terminator5/1
  Demux/2 -> Terminator6/1
  Demux/3 -> Discrete Delay Wing/1
  Discrete Delay Wing/1 -> Discrete Derivative/1, Reshape7/1
  Matrix Concatenate/1 -> V_Wg_wing1/1
  Demux1/2 -> Terminator4/1
  Discrete Derivative/1 -> Reshape8/1
  Constant/1 -> Reshape1/1
  Demux1/3 -> Terminator/1
  Demux1/1 -> Terminator3/1
  Matrix Concatenate1/1 -> V_Wg_dt_wing1/1
  Demux2/1 -> Terminator7/1
  Demux2/2 -> Terminator8/1
  Demux2/3 -> Discrete Delay HTP/1
  Discrete Delay HTP/1 -> Discrete Derivative1/1, Reshape5/1
  Matrix Concatenate2/1 -> V_Wg_wing2/1
  Constant1/1 -> Reshape2/1
  Discrete Derivative1/1 -> Reshape6/1
  Demux3/3 -> Terminator2/1
  Demux3/2 -> Terminator10/1
  Demux3/1 -> Terminator9/1
  Matrix Concatenate3/1 -> V_Wg_dt_wing2/1
  Demux4/1 -> Terminator11/1
  Demux4/2 -> Terminator12/1
  Demux4/3 -> Discrete Delay VTP/1
  Matrix Concatenate4/1 -> V_Wg_wing3/1
  Demux5/2 -> Terminator14/1
  Demux5/1 -> Terminator13/1
  Demux5/3 -> Terminator1/1
  Discrete Delay VTP/1 -> Discrete Derivative2/1, Reshape9/1
  Matrix Concatenate5/1 -> V_Wg_dt_wing3/1
  Matrix Concatenate6/1 -> V_Wg_fuselage/1
  Demux6/3 -> Discrete Delay Fuse/1
  Demux6/1 -> Terminator15/1
  Demux6/2 -> Terminator16/1
  Constant3/1 -> Reshape4/1
  Discrete Delay Fuse/1 -> Reshape11/1
  Selector/1 -> Demux7/1
  Discrete Derivative2/1 -> Reshape10/1
  Constant2/1 -> Reshape3/1
  Reshape2/1 -> Matrix Concatenate3/1, Matrix Concatenate3/2, Matrix Concatenate2/2, Matrix Concatenate2/1
  Reshape1/1 -> Matrix Concatenate1/2, Matrix Concatenate1/1, Matrix Concatenate/2, Matrix Concatenate/1
  Reshape3/1 -> Matrix Concatenate5/2, Matrix Concatenate5/1, Matrix Concatenate4/2, Matrix Concatenate4/1
  Reshape4/1 -> Matrix Concatenate6/1, Matrix Concatenate6/2
  Reshape5/1 -> Matrix Concatenate2/3
  Reshape6/1 -> Matrix Concatenate3/3
  Reshape7/1 -> Matrix Concatenate/3
  Reshape8/1 -> Matrix Concatenate1/3
  Reshape9/1 -> Matrix Concatenate4/3
  Reshape10/1 -> Matrix Concatenate5/3
  Reshape11/1 -> Matrix Concatenate6/3

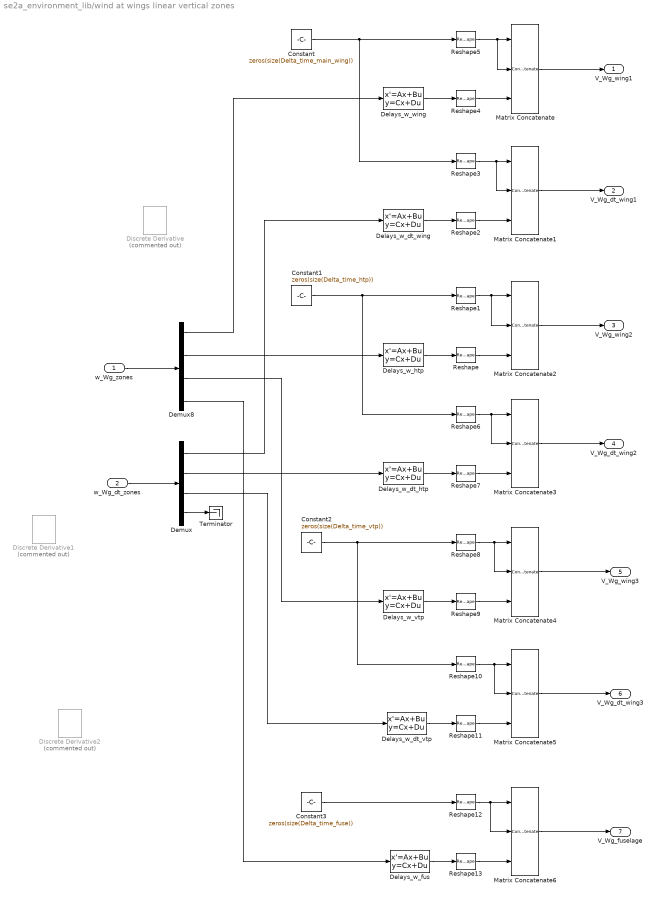
== system se2a_environment_lib/wind at wings linear vertical zones ==
  w_Wg_zones : Inport
  w_Wg_dt_zones : Inport  Port=2
  Constant : Constant  Value=zeros(size(Delta_time_main_wing))
  Constant1 : Constant  Value=zeros(size(Delta_time_htp))
  Constant2 : Constant  Value=zeros(size(Delta_time_vtp))
  Constant3 : Constant  Value=zeros(size(Delta_time_fuse))
  Delays_w_dt_htp : StateSpace  A=Delay_sys_htp.A  B=Delay_sys_htp.B  C=Delay_sys_htp.C  D=Delay_sys_htp.D  InitialCondition=0
  Delays_w_dt_vtp : StateSpace  A=Delay_sys_vtp.A  B=Delay_sys_vtp.B  C=Delay_sys_vtp.C  D=Delay_sys_vtp.D  InitialCondition=0
  Delays_w_dt_wing : StateSpace  A=Delay_sys_main_wing.A  B=Delay_sys_main_wing.B  C=Delay_sys_main_wing.C  D=Delay_sys_main_wing.D  InitialCondition=0
  Delays_w_fus : StateSpace  A=Delay_sys_fuse.A  B=Delay_sys_fuse.B  C=Delay_sys_fuse.C  D=Delay_sys_fuse.D  InitialCondition=0
  Delays_w_htp : StateSpace  A=Delay_sys_htp.A  B=Delay_sys_htp.B  C=Delay_sys_htp.C  D=Delay_sys_htp.D  InitialCondition=0
  Delays_w_vtp : StateSpace  A=Delay_sys_vtp.A  B=Delay_sys_vtp.B  C=Delay_sys_vtp.C  D=Delay_sys_vtp.D  InitialCondition=0
  Delays_w_wing : StateSpace  A=Delay_sys_main_wing.A  B=Delay_sys_main_wing.B  C=Delay_sys_main_wing.C  D=Delay_sys_main_wing.D  InitialCondition=0
  Demux : Demux
  Demux8 : Demux
  Discrete Derivative : simulink/Discrete/Discrete Derivative  Commented=on  gainval=1.0  ICPrevScaledInput=0.0  OutMin=[]  OutMax=[]  OutDataType=fixdt(1, 16)  OutScaling=2^-10  DoSatur=off
  Discrete Derivative1 : simulink/Discrete/Discrete Derivative  Commented=on  gainval=1.0  ICPrevScaledInput=0.0  OutMin=[]  OutMax=[]  OutDataType=fixdt(1, 16)  OutScaling=2^-10  DoSatur=off
  Discrete Derivative2 : simulink/Discrete/Discrete Derivative  Commented=on  gainval=1.0  ICPrevScaledInput=0.0  OutMin=[]  OutMax=[]  OutDataType=fixdt(1, 16)  OutScaling=2^-10  DoSatur=off
  Matrix Concatenate{,1..6} (7 alike) : Concatenate  NumInputs=3  Mode=Multidimensional array
  Reshape{,1..13} (14 alike) : Reshape  OutputDimensionality=Row vector (2-D)
  Terminator : Terminator
  V_Wg_wing1 : Outport
  V_Wg_dt_wing1 : Outport  Port=2
  V_Wg_wing2 : Outport  Port=3
  V_Wg_dt_wing2 : Outport  Port=4
  V_Wg_wing3 : Outport  Port=5
  V_Wg_dt_wing3 : Outport  Port=6
  V_Wg_fuselage : Outport  Port=7
  wires:
  Reshape13/1 -> Matrix Concatenate6/3
  Reshape12/1 -> Matrix Concatenate6/1, Matrix Concatenate6/2
  Reshape11/1 -> Matrix Concatenate5/3
  Reshape10/1 -> Matrix Concatenate5/2, Matrix Concatenate5/1
  Reshape9/1 -> Matrix Concatenate4/3
  Reshape8/1 -> Matrix Concatenate4/1, Matrix Concatenate4/2
  Reshape7/1 -> Matrix Concatenate3/3
  Reshape6/1 -> Matrix Concatenate3/2, Matrix Concatenate3/1
  Reshape5/1 -> Matrix Concatenate/2, Matrix Concatenate/1
  Reshape4/1 -> Matrix Concatenate/3
  Reshape3/1 -> Matrix Concatenate1/2, Matrix Concatenate1/1
  Reshape2/1 -> Matrix Concatenate1/3
  Reshape1/1 -> Matrix Concatenate2/2, Matrix Concatenate2/1
  Reshape/1 -> Matrix Concatenate2/3
  Demux8/1 -> Delays_w_wing/1
  Delays_w_wing/1 -> Reshape4/1
  Matrix Concatenate/1 -> V_Wg_wing1/1
  Delays_w_dt_wing/1 -> Reshape2/1
  Constant/1 -> Reshape5/1, Reshape3/1
  Matrix Concatenate1/1 -> V_Wg_dt_wing1/1
  Demux8/2 -> Delays_w_htp/1
  Delays_w_htp/1 -> Reshape/1
  Matrix Concatenate2/1 -> V_Wg_wing2/1
  Constant1/1 -> Reshape6/1, Reshape1/1
  Delays_w_dt_htp/1 -> Reshape7/1
  Matrix Concatenate3/1 -> V_Wg_dt_wing2/1
  Demux8/3 -> Delays_w_vtp/1
  Matrix Concatenate4/1 -> V_Wg_wing3/1
  Delays_w_vtp/1 -> Reshape9/1
  Matrix Concatenate5/1 -> V_Wg_dt_wing3/1
  Matrix Concatenate6/1 -> V_Wg_fuselage/1
  Demux8/4 -> Delays_w_fus/1
  Constant3/1 -> Reshape12/1
  Delays_w_fus/1 -> Reshape13/1
  Delays_w_dt_vtp/1 -> Reshape11/1
  Constant2/1 -> Reshape10/1, Reshape8/1
  w_Wg_zones/1 -> Demux8/1
  w_Wg_dt_zones/1 -> Demux/1
  Demux/1 -> Delays_w_dt_wing/1
  Demux/2 -> Delays_w_dt_htp/1
  Demux/3 -> Delays_w_dt_vtp/1
  Demux/4 -> Terminator/1

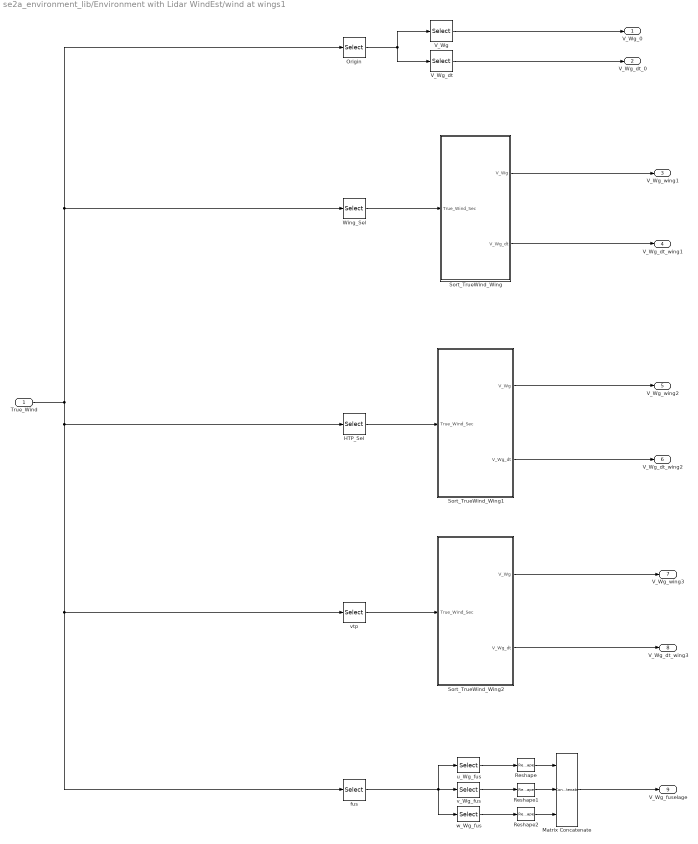
== system se2a_environment_lib/Environment with Lidar WindEst/wind at wings1 ==
  True_Wind : Inport
  HTP_Sel : Selector  InputPortWidth=size(Atmosphere.RequiredWindOutputs,1)  IndexOptions=Index vector (dialog)  Indices=(n_origin+6*n_wing+1):(n_origin+6*n_wing+6*n_htp)  OutputSizes=size(Atmosphere.RequiredWindOutputs,1)-3
  Matrix Concatenate : Concatenate  NumInputs=3  Mode=Multidimensional array
  Origin : Selector  InputPortWidth=size(Atmosphere.RequiredWindOutputs,1)  IndexOptions=Index vector (dialog)  Indices=[1:n_origin]  OutputSizes=1
  Reshape : Reshape  OutputDimensionality=Row vector (2-D)
  Reshape1 : Reshape  OutputDimensionality=Row vector (2-D)
  Reshape2 : Reshape  OutputDimensionality=Row vector (2-D)
  Sort_TrueWind_Wing : Subsystem  mask{n_wing=n_wing}
      mask prompts: n_wing "Number of section elements:"
  Sort_TrueWind_Wing1 : Subsystem  mask{n_wing=n_htp}
      mask prompts: n_wing "Number of section elements:"
  Sort_TrueWind_Wing2 : Subsystem  mask{n_wing=n_vtp}
      mask prompts: n_wing "Number of section elements:"
  V_Wg : Selector  InputPortWidth=n_origin  IndexOptions=Index vector (dialog)  Indices=[1:3]  OutputSizes=1
  V_Wg_dt : Selector  InputPortWidth=n_origin  IndexOptions=Index vector (dialog)  Indices=[4:6]  OutputSizes=1
  Wing_Sel : Selector  InputPortWidth=size(Atmosphere.RequiredWindOutputs,1)  IndexOptions=Index vector (dialog)  Indices=(n_origin+1):(n_origin+6*n_wing)  OutputSizes=size(Atmosphere.RequiredWindOutputs,1)-3
  fus : Selector  InputPortWidth=size(Atmosphere.RequiredWindOutputs,1)  IndexOptions=Index vector (dialog)  Indices=(n_origin+6*n_wing+6*n_htp+6*n_vtp+1):(n_origin+6*n_wing+6*n_htp+6*n_vtp+3*n_fus)  OutputSizes=size(Atmosphere.RequiredWindOutputs,1)-3
  u_Wg_fus : Selector  InputPortWidth=3*n_fus  IndexOptions=Index vector (dialog)  Indices=1:n_fus  OutputSizes=size(Atmosphere.RequiredWindOutputs,1)-3
  v_Wg_fus : Selector  InputPortWidth=3*n_fus  IndexOptions=Index vector (dialog)  Indices=(1+n_fus):(2*n_fus)  OutputSizes=size(Atmosphere.RequiredWindOutputs,1)-3
  vtp : Selector  InputPortWidth=size(Atmosphere.RequiredWindOutputs,1)  IndexOptions=Index vector (dialog)  Indices=(n_origin+6*n_wing+6*n_htp+1):(n_origin+6*n_wing+6*n_htp+6*n_vtp)  OutputSizes=size(Atmosphere.RequiredWindOutputs,1)-3
  w_Wg_fus : Selector  InputPortWidth=3*n_fus  IndexOptions=Index vector (dialog)  Indices=(1+2*n_fus):(3*n_fus)  OutputSizes=size(Atmosphere.RequiredWindOutputs,1)-3
  V_Wg_0 : Outport
  V_Wg_dt_0 : Outport  Port=2
  V_Wg_wing1 : Outport  Port=3
  V_Wg_dt_wing1 : Outport  Port=4
  V_Wg_wing2 : Outport  Port=5
  V_Wg_dt_wing2 : Outport  Port=6
  V_Wg_wing3 : Outport  Port=7
  V_Wg_dt_wing3 : Outport  Port=8
  V_Wg_fuselage : Outport  Port=9
  wires:
  Sort_TrueWind_Wing1/2(V_Wg_dt) -> V_Wg_dt_wing2/1
  Sort_TrueWind_Wing1/1(V_Wg) -> V_Wg_wing2/1
  True_Wind/1 -> vtp/1, fus/1, HTP_Sel/1, Origin/1, Wing_Sel/1
  Wing_Sel/1 -> Sort_TrueWind_Wing/1(True_Wind_Sec)
  Sort_TrueWind_Wing/1(V_Wg) -> V_Wg_wing1/1
  Sort_TrueWind_Wing/2(V_Wg_dt) -> V_Wg_dt_wing1/1
  HTP_Sel/1 -> Sort_TrueWind_Wing1/1(True_Wind_Sec)
  vtp/1 -> Sort_TrueWind_Wing2/1(True_Wind_Sec)
  Sort_TrueWind_Wing2/2(V_Wg_dt) -> V_Wg_dt_wing3/1
  Sort_TrueWind_Wing2/1(V_Wg) -> V_Wg_wing3/1
  Reshape2/1 -> Matrix Concatenate/3
  u_Wg_fus/1 -> Reshape/1
  Matrix Concatenate/1 -> V_Wg_fuselage/1
  fus/1 -> w_Wg_fus/1, v_Wg_fus/1, u_Wg_fus/1
  Reshape1/1 -> Matrix Concatenate/2
  v_Wg_fus/1 -> Reshape1/1
  w_Wg_fus/1 -> Reshape2/1
  Reshape/1 -> Matrix Concatenate/1
  Origin/1 -> V_Wg/1, V_Wg_dt/1
  V_Wg/1 -> V_Wg_0/1
  V_Wg_dt/1 -> V_Wg_dt_0/1

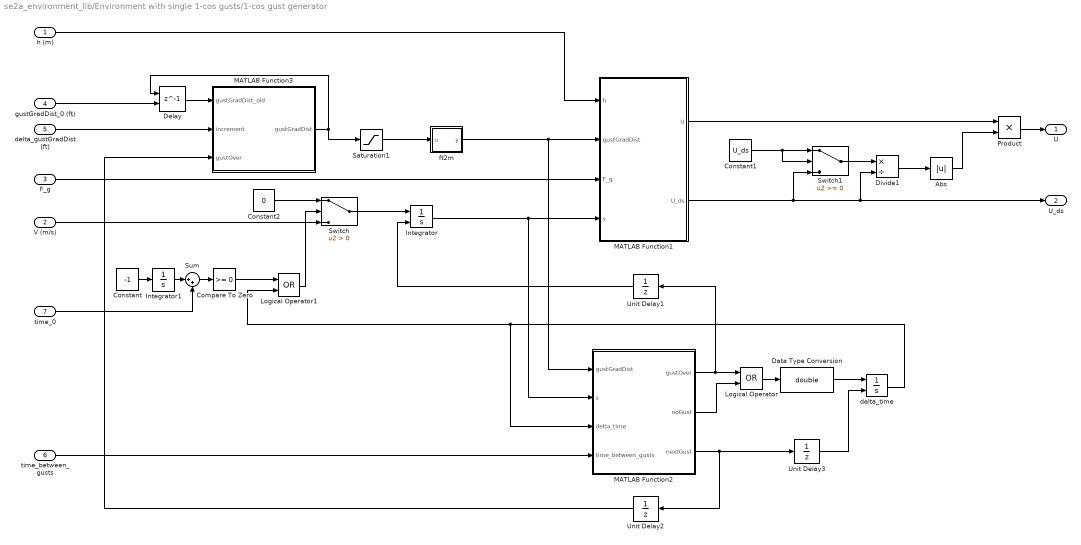
== system se2a_environment_lib/Environment with single 1-cos gusts/1-cos gust generator ==
  h (m) : Inport
  V (m/s) : Inport  Port=2
  F_g : Inport  Port=3
  gustGradDist_0 (ft) : Inport  Port=4
  delta_gustGradDist (ft) : Inport  Port=5
  time_between_gusts : Inport  Port=6
  time_0 : Inport  Port=7
  Abs : Abs
  Compare To Zero : simulink/Logic and Bit Operations/Compare To Zero  relop=>=  OutDataTypeStr=boolean
  Constant : Constant  Value=-1
  Constant1 : Constant  Value=U_ds
  Constant2 : Constant  Value=0
  Data Type Conversion : DataTypeConversion  OutDataTypeStr=double
  Delay : Delay  DelayLength=1  InitialConditionSource=Input port
      settings: InputPortMap=u0,p4
  Divide1 : Product  Inputs=*/
  Integrator : Integrator  ExternalReset=rising
  Integrator1 : Integrator
  Logical Operator : Logic  Operator=OR  AllPortsSameDT=off  OutDataTypeStr=boolean
  Logical Operator1 : Logic  Operator=OR  AllPortsSameDT=off  OutDataTypeStr=boolean
  MATLAB Function1 : MATLAB Function  TreatAsAtomicUnit=on
  MATLAB Function2 : MATLAB Function  TreatAsAtomicUnit=on
  MATLAB Function3 : MATLAB Function  TreatAsAtomicUnit=on
  Product : Product  Inputs=**
  Saturation1 : Saturate  UpperLimit=349.9  LowerLimit=30.1
  Sum : Sum  Inputs=|++
  Switch : Switch  Criteria=u2 > Threshold
  Switch1 : Switch
  Unit Delay1 : UnitDelay  SampleTime=-1
  Unit Delay2 : UnitDelay  SampleTime=-1
  Unit Delay3 : UnitDelay  SampleTime=-1
  delta_time : Integrator  ExternalReset=rising
  ft2m : MATLAB Function  TreatAsAtomicUnit=on
  U : Outport
  U_ds : Outport  Port=2
  wires:
  delta_gustGradDist (ft)/1 -> MATLAB Function3/2(increment)
  MATLAB Function1/1(U) -> Product/1
  Saturation1/1 -> ft2m/1(u)
  h (m)/1 -> MATLAB Function1/1(h)
  F_g/1 -> MATLAB Function1/3(F_g)
  MATLAB Function1/2(U_ds) -> Switch1/3, U_ds/1, Divide1/2
  ft2m/1(y) -> MATLAB Function1/2(gustGradDist), MATLAB Function2/1(gustGradDist)
  MATLAB Function3/1(gustGradDist) -> Saturation1/1, Delay/1
  Integrator/1 -> MATLAB Function1/4(s), MATLAB Function2/2(s)
  V (m/s)/1 -> Switch/3
  Switch/1 -> Integrator/1
  Constant2/1 -> Switch/1
  time_between_gusts/1 -> MATLAB Function2/4(time_between_gusts)
  MATLAB Function2/2(noGust) -> Logical Operator/2
  Logical Operator/1 -> Data Type Conversion/1
  MATLAB Function2/1(gustOver) -> Logical Operator/1, Unit Delay1/1
  MATLAB Function2/3(nextGust) -> Unit Delay3/1, Unit Delay2/1
  Data Type Conversion/1 -> delta_time/1
  Unit Delay1/1 -> Integrator/2
  Unit Delay2/1 -> MATLAB Function3/3(gustOver)
  delta_time/1 -> Logical Operator1/2, MATLAB Function2/3(delta_time)
  Unit Delay3/1 -> delta_time/2
  Delay/1 -> MATLAB Function3/1(gustGradDist_old)
  gustGradDist_0 (ft)/1 -> Delay/2
  Constant/1 -> Integrator1/1
  time_0/1 -> Sum/2
  Logical Operator1/1 -> Switch/2
  Integrator1/1 -> Sum/1
  Compare To Zero/1 -> Logical Operator1/1
  Sum/1 -> Compare To Zero/1
  Constant1/1 -> Switch1/1, Switch1/2
  Switch1/1 -> Divide1/1
  Divide1/1 -> Abs/1
  Product/1 -> U/1
  Abs/1 -> Product/2

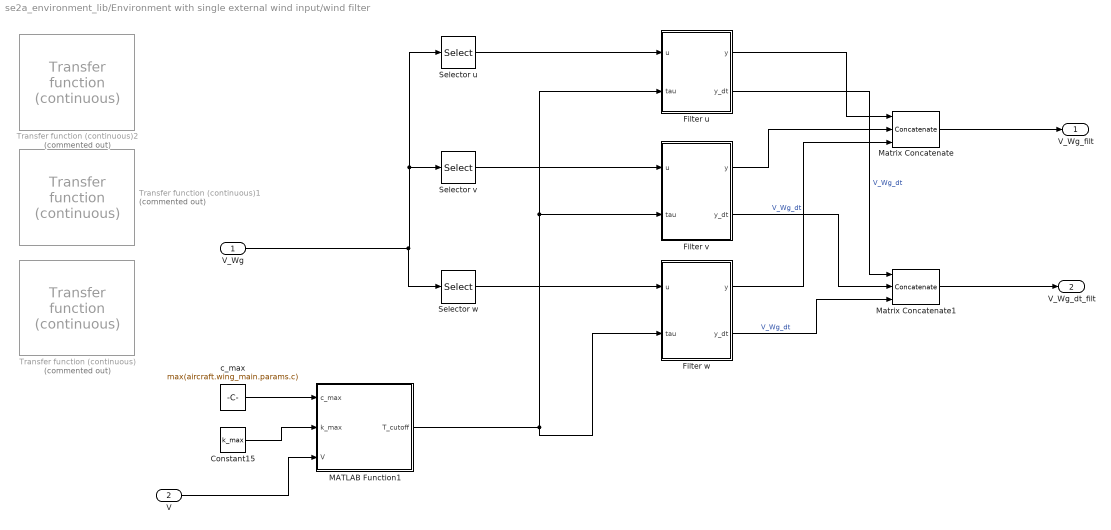
== system se2a_environment_lib/Environment with single external wind input/wind filter ==
  V_Wg : Inport
  V : Inport  Port=2
  Constant15 : Constant  Value=k_max
  Filter u : Subsystem
  Filter v : Subsystem
  Filter w : Subsystem
  MATLAB Function1 : MATLAB Function  TreatAsAtomicUnit=on
  Matrix Concatenate : Concatenate  NumInputs=3  Mode=Multidimensional array
  Matrix Concatenate1 : Concatenate  NumInputs=3  Mode=Multidimensional array
  Selector u : Selector  NumberOfDimensions=2  InputPortWidth=3  IndexOptions=Index vector (dialog),Select all  Indices=1,1  OutputSizes=1,1
  Selector v : Selector  NumberOfDimensions=2  InputPortWidth=3  IndexOptions=Index vector (dialog),Select all  Indices=2,1  OutputSizes=1,1
  Selector w : Selector  NumberOfDimensions=2  InputPortWidth=3  IndexOptions=Index vector (dialog),Select all  Indices=3,1  OutputSizes=1,1
  Transfer function (continuous) : linear_systems_lib/Transfer function (continuous)  Commented=on
      settings: SourceProductName=LADAC
  Transfer function (continuous)1 : linear_systems_lib/Transfer function (continuous)  Commented=on
      settings: SourceProductName=LADAC
  Transfer function (continuous)2 : linear_systems_lib/Transfer function (continuous)  Commented=on
      settings: SourceProductName=LADAC
  c_max : Constant  Value=max(aircraft.wing_main.params.c)
  V_Wg_filt : Outport
  V_Wg_dt_filt : Outport  Port=2
  wires:
  MATLAB Function1/1(T_cutoff) -> Filter w/2(tau), Filter u/2(tau), Filter v/2(tau)
  c_max/1 -> MATLAB Function1/1(c_max)
  V/1 -> MATLAB Function1/3(V)
  Filter w/1(y) -> Matrix Concatenate/3
  Constant15/1 -> MATLAB Function1/2(k_max)
  Filter w/2(y_dt) -> Matrix Concatenate1/3  "V_Wg_dt"
  Selector u/1 -> Filter u/1(u)
  Filter u/1(y) -> Matrix Concatenate/1
  Filter v/1(y) -> Matrix Concatenate/2
  Matrix Concatenate/1 -> V_Wg_filt/1
  Filter v/2(y_dt) -> Matrix Concatenate1/2  "V_Wg_dt"
  Filter u/2(y_dt) -> Matrix Concatenate1/1  "V_Wg_dt"
  Matrix Concatenate1/1 -> V_Wg_dt_filt/1
  V_Wg/1 -> Selector w/1, Selector u/1, Selector v/1
  Selector w/1 -> Filter w/1(u)
  Selector v/1 -> Filter v/1(u)

== system se2a_environment_lib/Environment with zonal external wind input linear/wind filter ==
  note: u_Wg, v_Wg always equal 0
  V_Wg : Inport
  V : Inport  Port=2
  Constant15 : Constant  Value=k_max
  Filter u : Subsystem  Commented=on
  Filter v : Subsystem  Commented=on
  Filter w : Subsystem
  MATLAB Function1 : MATLAB Function  TreatAsAtomicUnit=on
  Matrix Concatenate : Concatenate  NumInputs=3  Mode=Multidimensional array
  Matrix Concatenate1 : Concatenate  NumInputs=3  Mode=Multidimensional array
  Selector u : Selector  NumberOfDimensions=2  InputPortWidth=3  IndexOptions=Index vector (dialog),Select all  Indices=1,1  OutputSizes=1,1
  Selector v : Selector  NumberOfDimensions=2  InputPortWidth=3  IndexOptions=Index vector (dialog),Select all  Indices=2,1  OutputSizes=1,1
  Selector w : Selector  NumberOfDimensions=2  InputPortWidth=3  IndexOptions=Index vector (dialog),Select all  Indices=3,1  OutputSizes=1,1
  Transfer function (continuous) : linear_systems_lib/Transfer function (continuous)  Commented=on
      settings: SourceProductName=LADAC
  Transfer function (continuous)1 : linear_systems_lib/Transfer function (continuous)  Commented=on
      settings: SourceProductName=LADAC
  Transfer function (continuous)2 : linear_systems_lib/Transfer function (continuous)  Commented=on
      settings: SourceProductName=LADAC
  c_max : Constant  Value=max(aircraft.wing_main.params.c)
  V_Wg_filt : Outport
  V_Wg_dt_filt : Outport  Port=2
  wires:
  Selector w/1 -> Filter w/1(u)
  V_Wg/1 -> Selector v/1, Selector u/1, Selector w/1
  Matrix Concatenate1/1 -> V_Wg_dt_filt/1
  Selector u/1 -> Matrix Concatenate1/1, Matrix Concatenate/1  "V_Wg_dt"
  Selector v/1 -> Matrix Concatenate1/2, Matrix Concatenate/2  "V_Wg_dt"
  Matrix Concatenate/1 -> V_Wg_filt/1
  Filter w/2(y_dt) -> Matrix Concatenate1/3  "V_Wg_dt"
  Constant15/1 -> MATLAB Function1/2(k_max)
  Filter w/1(y) -> Matrix Concatenate/3
  V/1 -> MATLAB Function1/3(V)
  c_max/1 -> MATLAB Function1/1(c_max)
  MATLAB Function1/1(T_cutoff) -> Filter w/2(tau)
